simulink model "Active_Suspension_PID_Velocity_Test"  (R2025b)
settings: Solver=VariableStepAuto  StartTime=0.0  StopTime=2.5  RelTol=1e-3
values from neighbouring files (symbols this model uses):
  c_s = 2100    [Report_Script_Suspension.m]
  k_s = 28500    [Report_Script_Suspension.m]
  k_u = 200000    [Report_Script_Suspension.m]
  m_s = (m_veh*wbf*wbl) - m_u    (= 565.5)    [Report_Script_Suspension.m]
  m_u = m_uf    (= 45)    [Report_Script_Suspension.m]
  mph_to_ms = 0.44704    [Report_Script_Suspension.m]
  v_mph = 20    [Report_Script_Suspension.m]
undefined symbols (not defined in the file or in its folder): road_profile_change, road_surface_length
libraries: slpidlib x1
settings Model: Creator=jens.lahr  LastModifiedBy=M Wasib
settings ModelReferenceCC: EnableRefExpFcnMdlSchedulingChecks=on
settings RTWCC: GPUComputeCapability=3.5

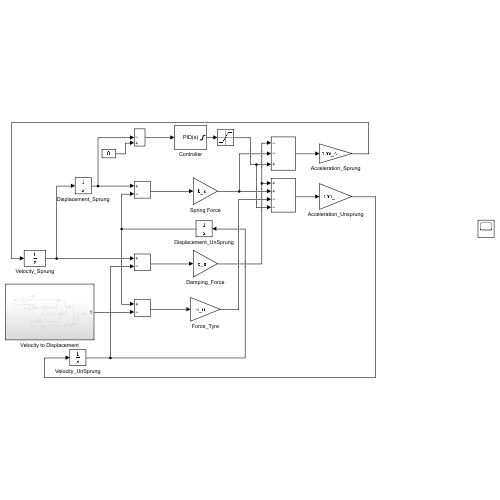
[thumbnail: Simulink's stored preview of the top-level diagram]
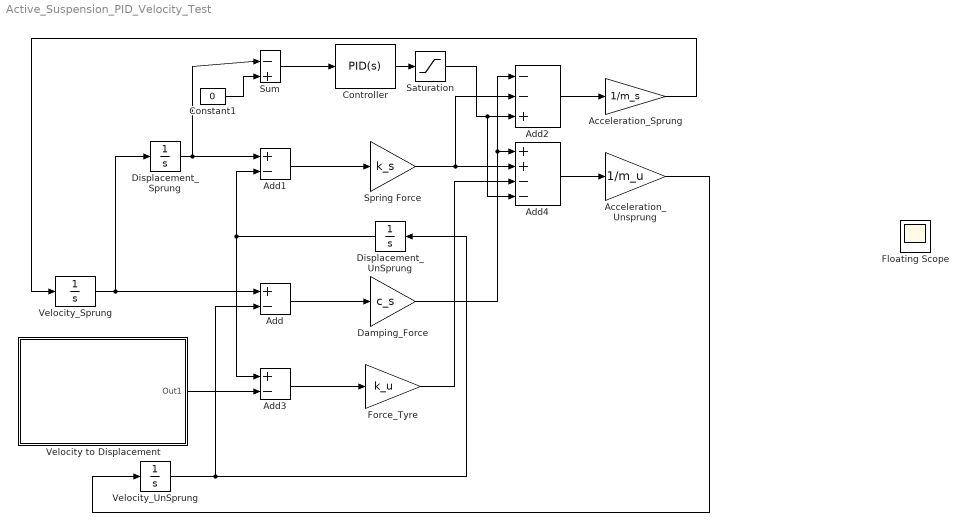
== system Active_Suspension_PID_Velocity_Test ==
  Acceleration_Sprung : Gain  Gain=1/m_s
  Acceleration_Unsprung : Gain  Gain=1/m_u
  Add : Sum  Inputs=+-
  Add1 : Sum  Inputs=+-
  Add2 : Sum  Inputs=--+
  Add3 : Sum  Inputs=+-
  Add4 : Sum  Inputs=++--
  Constant1 : Constant  Value=0
  Controller : slpidlib/PID Controller  Controller=PID  Form=Parallel  TimeDomain=Continuous-time  UseExternalTs=off  SampleTime=-1  IntegratorMethod=Forward Euler  FilterMethod=Forward Euler  ControllerParametersSource=internal  P=350  I=0  UseKiTs=off  D=10000  UseExternalDerivativeSource=off  N=500  UseFilter=on  TunerSelectOption=Transfer Function Based (PID Tuner App)  InitialConditionSource=internal  InitialConditionForIntegrator=0  InitialConditionForFilter=0  DifferentiatorICPrevScaledInput=0  ExternalReset=none  TrackingMode=off  Kt=1  LimitOutput=on  SatLimitsSource=internal  UpperSaturationLimit=1000000  LowerSaturationLimit=-1000000  LinearizeAsGain=on  AntiWindupMode=none  Kb=1  LimitIntegrator=off  UpperIntegratorSaturationLimit=inf  LowerIntegratorSaturationLimit=-inf  POutMin=[]  POutMax=[]  IOutMin=[]  IOutMax=[]  DOutMin=[]  DOutMax=[]  NOutMin=[]  NOutMax=[]  SumOutMin=[]  SumOutMax=[]  SaturationOutMin=[]  SaturationOutMax=[]  PParamMin=[]  PParamMax=[]  IParamMin=[]  IParamMax=[]  DParamMin=[]  DParamMax=[]  NParamMin=[]  NParamMax=[]  KbParamMin=[]  KbParamMax=[]  KtParamMin=[]  KtParamMax=[]  KbOutMin=[]  KbOutMax=[]  KtOutMin=[]  KtOutMax=[]  IntegratorOutMin=[]  IntegratorOutMax=[]  FilterOutMin=[]  FilterOutMax=[]  SumI1OutMin=[]  SumI1OutMax=[]  SumI2OutMin=[]  SumI2OutMax=[]  SumI3OutMin=[]  SumI3OutMax=[]  SumI4OutMin=[]  SumI4OutMax=[]  SumDOutMin=[]  SumDOutMax=[]  DifferentiatorOutMin=[]  DifferentiatorOutMax=[]  FilterDiffOutCoefMin=[]  FilterDiffOutCoefMax=[]  ReciprocalOutMin=[]  ReciprocalOutMax=[]  SumDenOutMin=[]  SumDenOutMax=[]  SumNumOutMin=[]  SumNumOutMax=[]  DivideOutMin=[]  DivideOutMax=[]  UdiffTsProdOutMin=[]  UdiffTsProdOutMax=[]  NTsProdOutMin=[]  NTsProdOutMax=[]  UintegralTsProdOutMin=[]  UintegralTsProdOutMax=[]  UngainTsProdOutMin=[]  UngainTsProdOutMax=[]  ClampingZeroOutDataTypeStr=Inherit: Inherit via back propagation  ClampingZeroOutMin=[]  ClampingZeroOutMax=[]  FilterDenConstantOutDataTypeStr=Inherit: Inherit via back propagation  FilterDenConstantOutMin=[]  FilterDenConstantOutMax=[]  PCopyOutDataTypeStr=Inherit: Inherit via back propagation  PCopyOutMin=[]  PCopyOutMax=[]  NCopyOutDataTypeStr=Inherit: Inherit via back propagation  NCopyOutMin=[]  NCopyOutMax=[]  IntegratorContinuousStateAttributes=''  IntegratorStateMustResolveToSignalObject=off  IntegratorRTWStateStorageClass=Auto  FilterContinuousStateAttributes=''  FilterStateMustResolveToSignalObject=off  FilterRTWStateStorageClass=Auto  ParallelPVariant=InternalParameters  IdealPVariant=Disabled  IVariant=InternalParameters  DVariant=InternalParameters  IntegratorVariant=Continuous  SatVariant=Enabled  AWVariant=Passthrough  PCopyVariant=Disabled  TRVariant=Disabled  FdbkBlocksVariant=Forward  IdealPFdbkVariant=Disabled  SatFdbkVariant=Disabled  DerivativeFilterVariant=ContFilter  NVariant=InternalParameters  NCopyVariant=Disabled  FilterICVariant=InternalICsFilter  IntegratorICVariant=InternalICs  ExternalResetVariant=Disabled  TRSumVariant=Passthrough  SumFdbkVariant=Disabled  SumVariant=Sum_PID  TsampFilterVariant=InternalTs  TsampNgainVariant=Passthrough  TsampIntegralVariant=Disabled_SignalSpec  ExternalSaturationOutDataTypeStr=Inherit: Same as second input  DerivativeSourceVariant=ErrorSignal  PreIntVariant=InternalPreInt
  Damping_Force : Gain  Gain=c_s
  Displacement_Sprung : Integrator
  Displacement_UnSprung : Integrator
  Floating Scope : Scope
      settings: IsFloating=on  Floating=on  ActiveDisplayYMinimum=-0.0016538104770371317  ActiveDisplayYMaximum=0.0025014950303705531  DataLoggingVariableName=ScopeData5
  Force_Tyre : Gain  Gain=k_u
  Saturation : Saturate  UpperLimit=1500  LowerLimit=-1500
  Spring Force : Gain  Gain=k_s
  Sum : Sum  Inputs=|-+
  Velocity to Displacement : Subsystem
  Velocity_Sprung : Integrator
  Velocity_UnSprung : Integrator
  wires:
  Add1/1 -> Spring Force/1
  Spring Force/1 -> Add4/2, Add2/2
  Sum/1 -> Controller/1
  Add3/1 -> Force_Tyre/1
  Velocity_Sprung/1 -> Displacement_Sprung/1, Add/1
  Velocity_UnSprung/1 -> Add/2, Displacement_UnSprung/1
  Constant1/1 -> Sum/2
  Displacement_Sprung/1 -> Add1/1, Sum/1
  Velocity to Displacement/1(Out1) -> Add3/2
  Add/1 -> Damping_Force/1
  Displacement_UnSprung/1 -> Add3/1, Add1/2
  Damping_Force/1 -> Add4/1, Add2/1
  Force_Tyre/1 -> Add4/3
  Acceleration_Sprung/1 -> Velocity_Sprung/1
  Add2/1 -> Acceleration_Sprung/1
  Add4/1 -> Acceleration_Unsprung/1
  Acceleration_Unsprung/1 -> Velocity_UnSprung/1
  Controller/1 -> Saturation/1
  Saturation/1 -> Add2/3, Add4/4

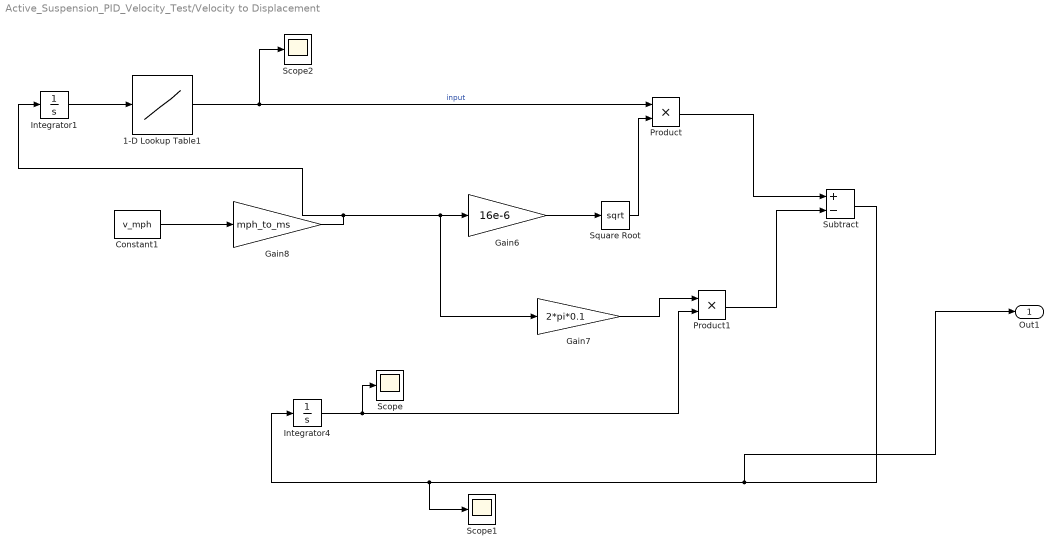
== system Active_Suspension_PID_Velocity_Test/Velocity to Displacement ==
  1-D Lookup Table1 : Lookup_n-D  NumberOfTableDimensions=1  BreakpointsForDimension1=road_surface_length  Table=road_profile_change  InternalRulePriority=Speed  RndMeth=Simplest
  Constant1 : Constant  Value=v_mph
  Gain6 : Gain  Gain=16e-6
  Gain7 : Gain  Gain=2*pi*0.1
  Gain8 : Gain  Gain=mph_to_ms
  Integrator1 : Integrator
  Integrator4 : Integrator
  Product : Product
  Product1 : Product
  Scope : Scope
      settings: ActiveDisplayYMinimum=-5E-5  ActiveDisplayYMaximum=0.00035
  Scope1 : Scope
      settings: ActiveDisplayYMinimum=-0.00258  ActiveDisplayYMaximum=0.00625  DataLoggingVariableName=ScopeData2
  Scope2 : Scope
      settings: ActiveDisplayYMinimum=-0.02992  ActiveDisplayYMaximum=0.16999  DataLoggingVariableName=ScopeData3
  Square Root : Sqrt
  Subtract : Sum  Inputs=+-
  Out1 : Outport
  wires:
  1-D Lookup Table1/1 -> Scope2/1, Product/1  "input"
  Product/1 -> Subtract/1
  Integrator4/1 -> Scope/1, Product1/2
  Subtract/1 -> Integrator4/1, Scope1/1, Out1/1
  Constant1/1 -> Gain8/1
  Product1/1 -> Subtract/2
  Square Root/1 -> Product/2
  Gain6/1 -> Square Root/1
  Gain7/1 -> Product1/1
  Gain8/1 -> Integrator1/1, Gain7/1, Gain6/1
  Integrator1/1 -> 1-D Lookup Table1/1
